simulink model "GlidePathControl_GlideSlopeDistance"  (R2018b)
settings: Solver=VariableStepAuto  StartTime=0.0  StopTime=20  RelTol=1e-3
libraries: simulink x1
settings Model: Creator=cdjsd  LastModifiedBy=cdjsd

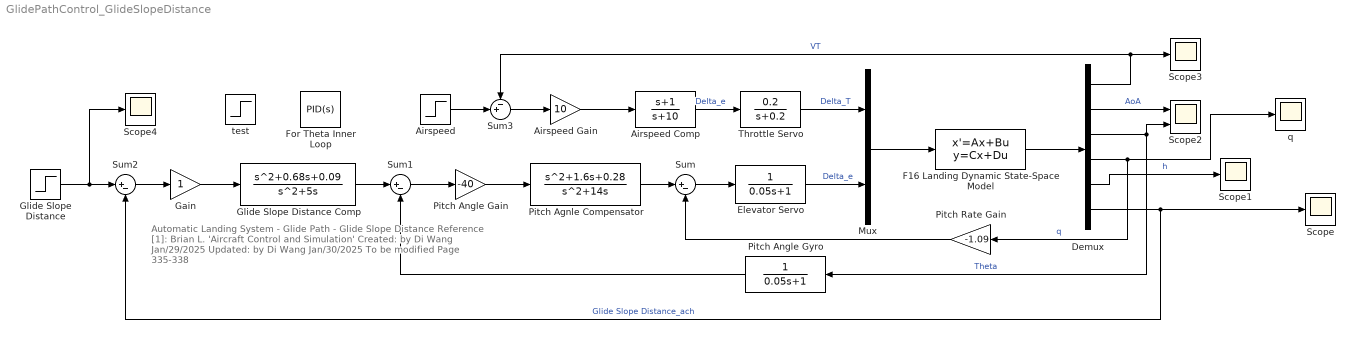
== system GlidePathControl_GlideSlopeDistance ==
  note: Automatic Landing System - Glide Path - Glide Slope Distance
      | Reference [1]: Brian L. 'Aircraft Control and Simulation'
      | Created: by Di Wang Jan/29/2025
      | Updated: by Di Wang Jan/30/2025
      | To be modified
      | Page 335-338
  Airspeed : Step  After=250  SampleTime=0
  Airspeed Comp : TransferFcn  Numerator=[1 1]  Denominator=[1 10]
  Airspeed Gain : Gain  Gain=10
  Demux : Demux  Outputs=6
  Elevator Servo : TransferFcn  Denominator=[0.05 1]
  F16 Landing Dynamic State-Space Model : StateSpace  A=|  B=[10.1 0; -1.5446e-4 0; 0 0; 0.024656 -0.01077; 0 0; 0 0]  C=[1 0 0 0 0 0; 0 57.296 0 0 0 0; 0 0 57.296 0 0 0; 0 0 0 57.296 0 0;0 0 0 0 1 0;0 0 0 0 0 1]  D=zeros(6,2)  InitialCondition=0
      | [-0.03858 18.984 -32.139 0 1.3233e-4 0;
      |      -0.001028 -0.63253 0.0056129 1 3.7553e-6 0;
      |      0 0 0 1 0 0;
      |      7.8601e-5 -0.75905 -0.00079341 -0.5183 -3.0808e-7 0;
      |      -0.04362 -249.76 249.76 0 0 0;
      |      0 -250 250 0 0 0]
  For Theta Inner Loop : simulink/Continuous/PID Controller  Controller=PID  Form=Parallel  TimeDomain=Continuous-time  SampleTime=-1  IntegratorMethod=Forward Euler  FilterMethod=Forward Euler  ControllerParametersSource=internal  P=-11.2524593283904  I=-4.27404125765141  D=-7.34039041594789  UseFilter=on  N=517.712076224405  TunerSelectOption=Transfer Function Based (PID Tuner App)  InitialConditionSource=internal  InitialConditionForIntegrator=0  InitialConditionForFilter=0  DifferentiatorICPrevScaledInput=0  ExternalReset=none  TrackingMode=off  Kt=1  LimitOutput=off  UpperSaturationLimit=inf  LowerSaturationLimit=-inf  LinearizeAsGain=on  AntiWindupMode=none  Kb=1  POutMin=[]  POutMax=[]  IOutMin=[]  IOutMax=[]  DOutMin=[]  DOutMax=[]  NOutMin=[]  NOutMax=[]  SumOutMin=[]  SumOutMax=[]  SaturationOutMin=[]  SaturationOutMax=[]  PParamMin=[]  PParamMax=[]  IParamMin=[]  IParamMax=[]  DParamMin=[]  DParamMax=[]  NParamMin=[]  NParamMax=[]  KbParamMin=[]  KbParamMax=[]  KtParamMin=[]  KtParamMax=[]  KbOutMin=[]  KbOutMax=[]  KtOutMin=[]  KtOutMax=[]  IntegratorOutMin=[]  IntegratorOutMax=[]  FilterOutMin=[]  FilterOutMax=[]  SumI1OutMin=[]  SumI1OutMax=[]  SumI2OutMin=[]  SumI2OutMax=[]  SumI3OutMin=[]  SumI3OutMax=[]  SumI4OutMin=[]  SumI4OutMax=[]  SumDOutMin=[]  SumDOutMax=[]  DifferentiatorOutMin=[]  DifferentiatorOutMax=[]  FilterDiffOutCoefMin=[]  FilterDiffOutCoefMax=[]  ReciprocalOutMin=[]  ReciprocalOutMax=[]  SumDenOutMin=[]  SumDenOutMax=[]  SumNumOutMin=[]  SumNumOutMax=[]  DivideOutMin=[]  DivideOutMax=[]  IntegratorContinuousStateAttributes=''  IntegratorStateMustResolveToSignalObject=off  IntegratorRTWStateStorageClass=Auto  FilterContinuousStateAttributes=''  FilterStateMustResolveToSignalObject=off  FilterRTWStateStorageClass=Auto  ParallelPVariant=InternalParameters  IdealPVariant=Disabled  IVariant=InternalParameters  DVariant=InternalParameters  IntegratorVariant=Continuous  SatVariant=Disabled  AWVariant=Passthrough  PCopyVariant=Disabled  TRVariant=Disabled  FdbkBlocksVariant=Forward  IdealPFdbkVariant=Disabled  SatFdbkVariant=Disabled  DerivativeFilterVariant=ContFilter  NVariant=InternalParameters  NCopyVariant=Disabled  FilterICVariant=InternalICsFilter  IntegratorICVariant=InternalICs  ExternalResetVariant=Disabled  TRSumVariant=Passthrough  SumFdbkVariant=Disabled  SumVariant=Sum_PID
  Gain : Gain
  Glide Slope Distance : Step  Before=-1  After=0  SampleTime=0
  Glide Slope Distance Comp : TransferFcn  Numerator=[1 0.68 0.09]  Denominator=[1 5 0]
  Mux : Mux  Inputs=2
  Pitch Agnle Compensator : TransferFcn  Numerator=[1 1.6 0.28]  Denominator=[1 14 0]
  Pitch Angle Gain : Gain  Gain=-40
  Pitch Angle Gyro : TransferFcn  Denominator=[0.05 1]
  Pitch Rate Gain : Gain  Gain=-1.09
  Scope{,1,3..4} (4 alike) : Scope
  Scope2 : Scope  NumInputPorts=2
  Sum : Sum  Inputs=|+-
  Sum1 : Sum  Inputs=|+-
  Sum2 : Sum  Inputs=|+-
  Sum3 : Sum  Inputs=-+|
  Throttle Servo : TransferFcn  Numerator=[0.2]  Denominator=[1 0.2]
  q : Scope
  test : Step  SampleTime=0
  wires:
  Mux/1 -> F16 Landing Dynamic State-Space Model/1
  F16 Landing Dynamic State-Space Model/1 -> Demux/1
  Throttle Servo/1 -> Mux/1  "Delta_T"
  Elevator Servo/1 -> Mux/2  "Delta_e"
  Demux/1 -> Sum3/1, Scope3/1  "VT"
  Demux/2 -> Scope2/1  "AoA"
  Demux/3 -> Scope2/2, Pitch Angle Gyro/1  "Theta"
  Demux/4 -> Pitch Rate Gain/1, q/1  "q"
  Demux/5 -> Scope1/1  "h"
  Demux/6 -> Scope/1, Sum2/2  "Glide Slope Distance_ach"
  Sum/1 -> Elevator Servo/1
  Pitch Rate Gain/1 -> Sum/2
  Sum2/1 -> Gain/1
  Airspeed Comp/1 -> Throttle Servo/1  "Delta_e"
  Airspeed Gain/1 -> Airspeed Comp/1
  Sum3/1 -> Airspeed Gain/1
  Airspeed/1 -> Sum3/2
  Glide Slope Distance/1 -> Scope4/1, Sum2/1
  Pitch Angle Gyro/1 -> Sum1/2
  Sum1/1 -> Pitch Angle Gain/1
  Gain/1 -> Glide Slope Distance Comp/1
  Glide Slope Distance Comp/1 -> Sum1/1
  Pitch Angle Gain/1 -> Pitch Agnle Compensator/1
  Pitch Agnle Compensator/1 -> Sum/1
